simulink model "CSE1_Oculus_gesture"  (R2014a)
settings: Solver=ode4  StartTime=0.0  StopTime=inf  FixedStep=0.01  RelTol=1e-3
undefined symbols (not defined in the file): v_max
libraries: marine_gnc x11
(part 4 of 4)

== system CSE1_Oculus_gesture/Input/Guidance gains/Gesture guidance ==
  Mux4 : Mux  Inputs=3
  Mux5 : Mux  Inputs=3
  diag : MATLAB Function  TreatAsAtomicUnit=on
  diag1 : MATLAB Function  TreatAsAtomicUnit=on
  w_d_psi : S-Function  Priority=2  FunctionName=NIVeriStandIO  Parameters=width dtype portnum stime stype btype  EnableBusSupport=off  mask(NI VeriStand Inport){portnum=2, width=-1, stime=-1, dtype=auto, stype=auto, btype=1}
      mask prompts: portnum "Port number:"; width "Port dimensions (-1 for dynamically sized):"; stime "Sample time (-1 for inherited):"; dtype "Data type:"; stype "Signal type:"; btype "Block type:"
      mask help: Use this inport on any level of nested subsystems to allow NI VeriStand software to map signals to it.
      mask init:
      | NIVeriStandIO_init;
      settings: CopyFcn=NIVeriStand_MDL_functions('', 'IO_copy');  DeleteFcn=NIVeriStand_MDL_functions('', 'IO_delete');  MoveFcn=set_param(gcb, 'Mask', 'on');
      mask Callback portnum: NIVeriStand_MDL_functions('', 'IO_setportnum');
      mask TypeOptions dtype: auto | double | single | int8 | uint8 | int16 | uint16 | int32 | uint32 | boolean
      mask Callback dtype: NIVeriStand_MDL_functions('', 'IO_booleansignal');
      mask TypeOptions stype: auto | real | complex
      mask Display:
      | patch([-x x], [-y y], [.90980 .81960 .32156]);
      | plot([xrad -x x xrad], [yrad -y y yrad]);
      | fprintf('NI In%d', portnum);
  w_d_x : S-Function  Priority=3  FunctionName=NIVeriStandIO  Parameters=width dtype portnum stime stype btype  EnableBusSupport=off  mask(NI VeriStand Inport){portnum=3, width=-1, stime=-1, dtype=auto, stype=auto, btype=1}
      mask prompts: portnum "Port number:"; width "Port dimensions (-1 for dynamically sized):"; stime "Sample time (-1 for inherited):"; dtype "Data type:"; stype "Signal type:"; btype "Block type:"
      mask help: Use this inport on any level of nested subsystems to allow NI VeriStand software to map signals to it.
      mask init:
      | NIVeriStandIO_init;
      settings: CopyFcn=NIVeriStand_MDL_functions('', 'IO_copy');  DeleteFcn=NIVeriStand_MDL_functions('', 'IO_delete');  MoveFcn=set_param(gcb, 'Mask', 'on');
      mask Callback portnum: NIVeriStand_MDL_functions('', 'IO_setportnum');
      mask TypeOptions dtype: auto | double | single | int8 | uint8 | int16 | uint16 | int32 | uint32 | boolean
      mask Callback dtype: NIVeriStand_MDL_functions('', 'IO_booleansignal');
      mask TypeOptions stype: auto | real | complex
      mask Display:
      | patch([-x x], [-y y], [.90980 .81960 .32156]);
      | plot([xrad -x x xrad], [yrad -y y yrad]);
      | fprintf('NI In%d', portnum);
  w_d_y : S-Function  Priority=4  FunctionName=NIVeriStandIO  Parameters=width dtype portnum stime stype btype  EnableBusSupport=off  mask(NI VeriStand Inport){portnum=4, width=-1, stime=-1, dtype=auto, stype=auto, btype=1}
      mask prompts: portnum "Port number:"; width "Port dimensions (-1 for dynamically sized):"; stime "Sample time (-1 for inherited):"; dtype "Data type:"; stype "Signal type:"; btype "Block type:"
      mask help: Use this inport on any level of nested subsystems to allow NI VeriStand software to map signals to it.
      mask init:
      | NIVeriStandIO_init;
      settings: CopyFcn=NIVeriStand_MDL_functions('', 'IO_copy');  DeleteFcn=NIVeriStand_MDL_functions('', 'IO_delete');  MoveFcn=set_param(gcb, 'Mask', 'on');
      mask Callback portnum: NIVeriStand_MDL_functions('', 'IO_setportnum');
      mask TypeOptions dtype: auto | double | single | int8 | uint8 | int16 | uint16 | int32 | uint32 | boolean
      mask Callback dtype: NIVeriStand_MDL_functions('', 'IO_booleansignal');
      mask TypeOptions stype: auto | real | complex
      mask Display:
      | patch([-x x], [-y y], [.90980 .81960 .32156]);
      | plot([xrad -x x xrad], [yrad -y y yrad]);
      | fprintf('NI In%d', portnum);
  zeta_psi : S-Function  Priority=5  FunctionName=NIVeriStandIO  Parameters=width dtype portnum stime stype btype  EnableBusSupport=off  mask(NI VeriStand Inport){portnum=5, width=-1, stime=-1, dtype=auto, stype=auto, btype=1}
      mask prompts: portnum "Port number:"; width "Port dimensions (-1 for dynamically sized):"; stime "Sample time (-1 for inherited):"; dtype "Data type:"; stype "Signal type:"; btype "Block type:"
      mask help: Use this inport on any level of nested subsystems to allow NI VeriStand software to map signals to it.
      mask init:
      | NIVeriStandIO_init;
      settings: CopyFcn=NIVeriStand_MDL_functions('', 'IO_copy');  DeleteFcn=NIVeriStand_MDL_functions('', 'IO_delete');  MoveFcn=set_param(gcb, 'Mask', 'on');
      mask Callback portnum: NIVeriStand_MDL_functions('', 'IO_setportnum');
      mask TypeOptions dtype: auto | double | single | int8 | uint8 | int16 | uint16 | int32 | uint32 | boolean
      mask Callback dtype: NIVeriStand_MDL_functions('', 'IO_booleansignal');
      mask TypeOptions stype: auto | real | complex
      mask Display:
      | patch([-x x], [-y y], [.90980 .81960 .32156]);
      | plot([xrad -x x xrad], [yrad -y y yrad]);
      | fprintf('NI In%d', portnum);
  zeta_x : S-Function  Priority=6  FunctionName=NIVeriStandIO  Parameters=width dtype portnum stime stype btype  EnableBusSupport=off  mask(NI VeriStand Inport){portnum=6, width=-1, stime=-1, dtype=auto, stype=auto, btype=1}
      mask prompts: portnum "Port number:"; width "Port dimensions (-1 for dynamically sized):"; stime "Sample time (-1 for inherited):"; dtype "Data type:"; stype "Signal type:"; btype "Block type:"
      mask help: Use this inport on any level of nested subsystems to allow NI VeriStand software to map signals to it.
      mask init:
      | NIVeriStandIO_init;
      settings: CopyFcn=NIVeriStand_MDL_functions('', 'IO_copy');  DeleteFcn=NIVeriStand_MDL_functions('', 'IO_delete');  MoveFcn=set_param(gcb, 'Mask', 'on');
      mask Callback portnum: NIVeriStand_MDL_functions('', 'IO_setportnum');
      mask TypeOptions dtype: auto | double | single | int8 | uint8 | int16 | uint16 | int32 | uint32 | boolean
      mask Callback dtype: NIVeriStand_MDL_functions('', 'IO_booleansignal');
      mask TypeOptions stype: auto | real | complex
      mask Display:
      | patch([-x x], [-y y], [.90980 .81960 .32156]);
      | plot([xrad -x x xrad], [yrad -y y yrad]);
      | fprintf('NI In%d', portnum);
  zeta_y : S-Function  Priority=1  FunctionName=NIVeriStandIO  Parameters=width dtype portnum stime stype btype  EnableBusSupport=off  mask(NI VeriStand Inport){portnum=1, width=-1, stime=-1, dtype=auto, stype=auto, btype=1}
      mask prompts: portnum "Port number:"; width "Port dimensions (-1 for dynamically sized):"; stime "Sample time (-1 for inherited):"; dtype "Data type:"; stype "Signal type:"; btype "Block type:"
      mask help: Use this inport on any level of nested subsystems to allow NI VeriStand software to map signals to it.
      mask init:
      | NIVeriStandIO_init;
      settings: CopyFcn=NIVeriStand_MDL_functions('', 'IO_copy');  DeleteFcn=NIVeriStand_MDL_functions('', 'IO_delete');  MoveFcn=set_param(gcb, 'Mask', 'on');
      mask Callback portnum: NIVeriStand_MDL_functions('', 'IO_setportnum');
      mask TypeOptions dtype: auto | double | single | int8 | uint8 | int16 | uint16 | int32 | uint32 | boolean
      mask Callback dtype: NIVeriStand_MDL_functions('', 'IO_booleansignal');
      mask TypeOptions stype: auto | real | complex
      mask Display:
      | patch([-x x], [-y y], [.90980 .81960 .32156]);
      | plot([xrad -x x xrad], [yrad -y y yrad]);
      | fprintf('NI In%d', portnum);
  tag scope: w_d_2=global, zeta_2=global
  wires:
  diag/1(w_d) -> [w_d_2]
  Mux4/1 -> diag/1(w_d_vector)
  zeta_x/1 -> Mux5/1
  zeta_psi/1 -> Mux5/3
  zeta_y/1 -> Mux5/2
  Mux5/1 -> diag1/1(zeta_vector)
  diag1/1(Zeta) -> [zeta_2]
  w_d_x/1 -> Mux4/1
  w_d_y/1 -> Mux4/2
  w_d_psi/1 -> Mux4/3

== matlab function CSE1_Oculus_gesture/Guidance/Reference model/w_d^3 ==
  data: w_d input; y output
function y = fcn(w_d)
%#codegen

y = w_d^3;

== matlab function CSE1_Oculus_gesture/Guidance/Reference model/w_d^-2 ==
  data: w_d input; y output
function y = fcn(w_d)
%#codegen

y = w_d^-2;

== matlab function CSE1_Oculus_gesture/Guidance/Reference model/w_d*w_d ==
  data: w_d input; y output
function y = fcn(w_d)
%#codegen

y = w_d*w_d;

== matlab function CSE1_Oculus_gesture/Guidance/Reference model/w_d*w_d1 ==
  data: w_d input; y output; zeta input
function y = fcn(w_d,zeta)
%#codegen

y = 2*zeta*w_d;

== matlab function CSE1_Oculus_gesture/Input/Guidance gains/DP guidance/diag ==
  data: w_d output; w_d_vector input
function w_d = fcn(w_d_vector)
%#codegen

w_d = diag(w_d_vector);

== matlab function CSE1_Oculus_gesture/Input/Guidance gains/DP guidance/diag1 ==
  data: Zeta output; zeta_vector input
function Zeta = fcn(zeta_vector)
%#codegen

Zeta = diag(zeta_vector);

== matlab function CSE1_Oculus_gesture/Guidance/Vel Reference model1/w_d*w_d ==
  data: w_d input; y output
function y = fcn(w_d)
%#codegen

y = w_d*w_d;

== matlab function CSE1_Oculus_gesture/Guidance/Vel Reference model1/w_d*w_d1 ==
  data: w_d input; y output; zeta input
function y = fcn(w_d,zeta)
%#codegen

y = 2*zeta*w_d;

== matlab function CSE1_Oculus_gesture/Thrust allocation/Thrust allocation ==
  data: X input; Y input; u_BT output; N input; u_VSP output; alpha_VSP output; VSP_on input; omega_VSP output
function [u_BT,u_VSP,alpha_VSP,omega_VSP]= fcn(X,Y,N, VSP_on)

% Forces and moments vector
tau = [X
       Y
       N];

% Extended thrust configuration matrix
l_VSP = -0.4575;
l_BT  = 0.3875;
T = [1 0     0
     0 1     1
     0 l_VSP l_BT];

% Extended thrust coefficient matrix
F_max_VSP = 1.165;
F_max_BT  = 2.629;
K = [F_max_VSP 0         0
     0         F_max_VSP 0
     0         0         F_max_BT];

% tau = T*K*u inverse
u = K\(T\tau);

u_BT      = u(3);

u_VSP_x   = u(1);
u_VSP_y   = u(2);
u_VSP     = sqrt(u_VSP_x^2 + u_VSP_y^2);
alpha_VSP = atan2(u_VSP_y,u_VSP_x);

if VSP_on
    omega_VSP = 0.3;
else
    omega_VSP = 0;
end

== matlab function CSE1_Oculus_gesture/Guidance/Vel Reference model1/w_d^-2 ==
  data: w_d input; y output
function y = fcn(w_d)
%#codegen

y = w_d^-2;

== matlab function CSE1_Oculus_gesture/ctrl_out/Switch_subsystem/Switch_function ==
  data: Cross input; switch_signal output; Square input; Circle input; Triangle input; temp input
%% Function that takes in impulse button sigals [0,1] and sends out a 
% different signal depentent pn which button has been pressed

function switch_signal = fcn(Cross,Square,Circle,Triangle,temp)
%#codegen
persistent signal;

signal = temp;

if Cross ~= 0
    signal = 1;
end

if Square ~= 0
    signal = 2;
end

if Circle ~= 0
    signal = 3;
end
    
if Triangle ~= 0
    signal = 4; 
end

switch_signal = signal;

== matlab function CSE1_Oculus_gesture/ctrl_out/control limit checking ==
  data: u input; fault output
function fault= fcn(u)
u_BT       = u(1);
u_VSP1     = u(2);
u_VSP2     = u(3);
alpha_VSP1 = u(4);
alpha_VSP2 = u(5);
omega_VSP1 = u(6);
omega_VSP2 = u(7);

OK = -1  <= u_BT       & u_BT       <= 1  & ...
     0   <= u_VSP1     & u_VSP1     <= 1  & ...
     0   <= u_VSP1     & u_VSP1     <= 2  & ...
     -pi <= alpha_VSP1 & alpha_VSP1 <= pi & ...
     -pi <= alpha_VSP2 & alpha_VSP2 <= pi & ...
     -1  <= omega_VSP1 & omega_VSP1 <= 1  & ...
     -1  <= omega_VSP2 & omega_VSP2 <= 1  ;
 
fault = ~OK;

== matlab function CSE1_Oculus_gesture/ctrl_out/indicator/C ==
  data: switch_signal input; ctrl_student output; ctrl_DP_basic output; ctrl_sixaxis2force output; ctrl_sixaxis2thruster output
function [ctrl_student,ctrl_DP_basic,ctrl_sixaxis2force,ctrl_sixaxis2thruster]= fcn(switch_signal)

ctrl_sixaxis2thruster = false;
ctrl_sixaxis2force    = false;
ctrl_DP_basic         = false;
ctrl_student          = false;

if switch_signal     == 1
    ctrl_student          = true; 
elseif switch_signal == 2
    ctrl_sixaxis2force    = true; 
elseif switch_signal == 3
    ctrl_DP_basic         = true; 
elseif switch_signal == 4
    ctrl_sixaxis2thruster = true;
else
    
end

== matlab function CSE1_Oculus_gesture/Input/Gesture based ctrl/MATLAB Function ==
  data: roll input; Roll output; pitch input; yaw input; Pitch output; Yaw output
function [Roll, Pitch, Yaw] = fcn(roll,pitch,yaw)
%#codegen
if abs(roll) < 5*2/180
    Roll = 0;
else
    Roll = roll;
end

if abs(pitch) < 5*2/180
    Pitch = 0;
else
    Pitch = pitch;
end

if abs(yaw) < 5*2/180
    Yaw = 0;
else
    Yaw = yaw;
end

== matlab function CSE1_Oculus_gesture/Input/Control Gains/MATLAB Function ==
  data: K_p output; K_p1 input
function K_p = fcn(K_p1)
%#codegen

K_p = diag(K_p1);

== matlab function CSE1_Oculus_gesture/Input/Control Gains/MATLAB Function1 ==
  data: K_i output; K_i1 input
function K_i = fcn(K_i1)
%#codegen

K_i = diag(K_i1);

== matlab function CSE1_Oculus_gesture/Input/Control Gains/MATLAB Function2 ==
  data: K_d output; K_d1 input
function K_d = fcn(K_d1)
%#codegen

K_d = diag(K_d1);

== matlab function CSE1_Oculus_gesture/Output/diag2vector ==
  data: u input; y output
function y = fcn(u)
%#codegen

y = [u(1,1),u(2,2),u(3,3)]';

== matlab function CSE1_Oculus_gesture/Output/diag2vector1 ==
  data: u input; y output
function y = fcn(u)
%#codegen

y = [u(1,1),u(2,2),u(3,3)]';

== matlab function CSE1_Oculus_gesture/Input/Guidance gains/Gesture guidance/diag ==
  data: w_d output; w_d_vector input
function w_d = fcn(w_d_vector)
%#codegen

w_d = diag(w_d_vector);

== matlab function CSE1_Oculus_gesture/Input/Guidance gains/Gesture guidance/diag1 ==
  data: Zeta output; zeta_vector input
function Zeta = fcn(zeta_vector)
%#codegen

Zeta = diag(zeta_vector);

== matlab function CSE1_Oculus_gesture/Output/diag2vector2 ==
  data: u input; y output
function y = fcn(u)
%#codegen

y = [u(1,1),u(2,2),u(3,3)]';

== matlab function CSE1_Oculus_gesture/Output/diag2vector3 ==
  data: u input; y output
function y = fcn(u)
%#codegen

y = [u(1,1),u(2,2),u(3,3)]';

== matlab function CSE1_Oculus_gesture/Output/diag2vector4 ==
  data: u input; y output
function y = fcn(u)
%#codegen

y = [u(1,1),u(2,2),u(3,3)]';

== matlab function CSE1_Oculus_gesture/Navigation /Derivative filter/MATLAB Function ==
  data: a input; eta_filtered output; eta input; eta_filtered_prev input
function eta_filtered = fcn(a,eta,eta_filtered_prev)

eta_filtered = a*eta + (1-a)*eta_filtered_prev;

== matlab function CSE1_Oculus_gesture/Navigation /Derivative filter/MATLAB Function1 ==
  data: h input; eta_dot output; eta input; eta_prev input
function eta_dot = fcn(h,eta,eta_prev)

eta_dot = (eta-eta_prev)./h;

== matlab function CSE1_Oculus_gesture/Navigation /Derivative filter/MATLAB Function2 ==
  data: a input; eta_dot_filtered output; eta_dot input; eta_dot_filtered_prev input
function eta_dot_filtered = fcn(a,eta_dot,eta_dot_filtered_prev)

eta_dot_filtered = a*eta_dot + (1-a)*eta_dot_filtered_prev;

== matlab function CSE1_Oculus_gesture/Navigation /Derivative filter/MATLAB Function3 ==
  data: eta_dot input; nu output; psi input
function nu = fcn(eta_dot,psi)

R_inv = [cos(psi)  sin(psi) 0
         -sin(psi) cos(psi) 0
         0         0        1];
nu = R_inv*eta_dot;

== matlab function CSE1_Oculus_gesture/Guidance/Vel Reference model1/w_d^3 ==
  data: w_d input; y output
function y = fcn(w_d)
%#codegen

y = w_d^3;

== matlab function CSE1_Oculus_gesture/Input/Gesture based ctrl/MATLAB Function4 ==
  data: K_p output; K_p1 input
function K_p = fcn(K_p1)
%#codegen

K_p = diag(K_p1);
